simulink model "TestPath"  (R2022b)
settings: Solver=VariableStepAuto  StartTime=0.0  StopTime=1  RelTol=1e-3
settings Model: Creator=ADMIN  LastModifiedBy=ADMIN

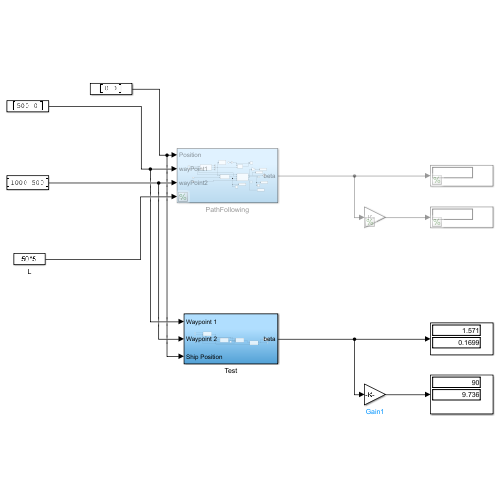
[thumbnail: Simulink's stored preview of the top-level diagram]
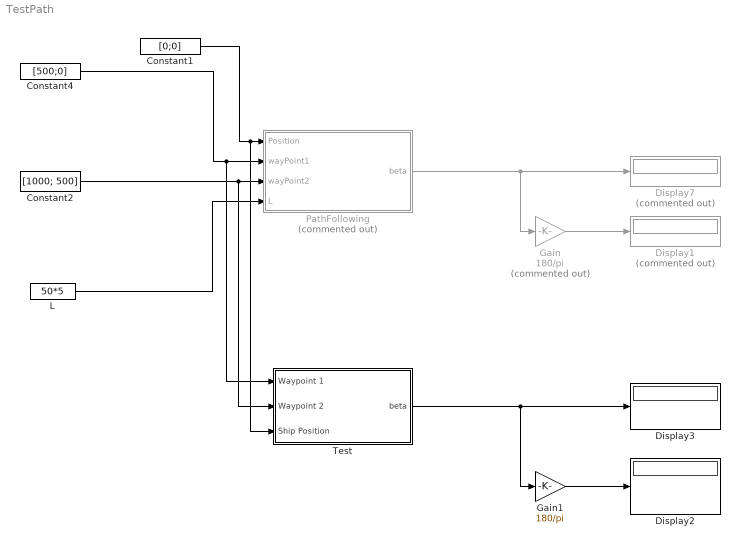
== system TestPath ==
  Constant1 : Constant  Value=[0;0]
  Constant2 : Constant  Value=[1000; 500]
  Constant4 : Constant  Value=[500;0]
  Display1 : Display  Commented=on
  Display2 : Display
  Display3 : Display
  Display7 : Display  Commented=on
  Gain : Gain  Commented=on  Gain=180/pi
  Gain1 : Gain  Gain=180/pi
  L : Constant  Value=50*5
  PathFollowing : Subsystem  Commented=on
  Test : Subsystem
  wires:
  PathFollowing/1(beta) -> Gain/1, Display7/1
  Constant2/1 -> PathFollowing/3(wayPoint2), Test/2(Waypoint 2)
  L/1 -> PathFollowing/4(L)
  Constant4/1 -> PathFollowing/2(wayPoint1), Test/1(Waypoint 1)
  Constant1/1 -> Test/3(Ship Position), PathFollowing/1(Position)
  Gain/1 -> Display1/1
  Gain1/1 -> Display2/1
  Test/1(beta) -> Display3/1, Gain1/1

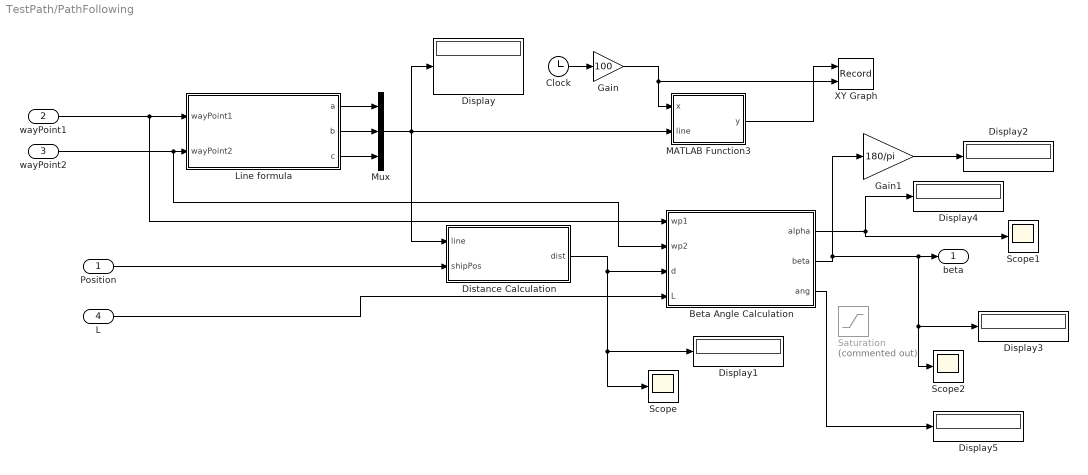
== system TestPath/PathFollowing ==
  Position : Inport
  wayPoint1 : Inport  Port=2
  wayPoint2 : Inport  Port=3
  L : Inport  Port=4
  Beta Angle Calculation : MATLAB Function  TreatAsAtomicUnit=on
  Clock : Clock
  Display{,1..5} (6 alike) : Display
  Distance Calculation : MATLAB Function  TreatAsAtomicUnit=on
  Gain : Gain  Gain=100
  Gain1 : Gain  Gain=180/pi
  Line formula : MATLAB Function  TreatAsAtomicUnit=on
  MATLAB Function3 : MATLAB Function  TreatAsAtomicUnit=on
  Mux : Mux  Inputs=3
  Saturation : Saturate  Commented=on
  Scope : Scope
  Scope1 : Scope
  Scope2 : Scope
  XY Graph : Record  FileSettingsInternal="{\"entries\":[{\"content\":{\"excelSettings\":{\"content\":{},\"type\":\"Streamout.ExcelSettings\"}},\"type\":\"Streamout.FileSettingStorage\",\"uuid\":\"7b3461a9-4dfd-4a0d-8e09-ea25a3eef10c\"}],\"packageUris\":[\"http://schema.mathworks.com/mf0/streamout_blocks/R2020a\"],\"version\":\"1.0\"}"  Layout=[1 1]  SignalsInternal="{\"entries\":[{\"content\":{\"signals\":[{\"content\":{\"blockPath\":[\"TestPath/PathFollowing/XY Graph\"],\"channel\":[],\"dimensions\":[1],\"domain\":\"TestPath/PathFollowing/XY Graph\",\"lineColor\":\"#64d413\",\"plots\":[1],\"port\":1,\"sid\":[],\"signalID\":197,\"signalName\":\"MATLAB Function3\"},\"type\":\"RecordBlkView.Signal\",\"uuid\":\"7b2fa58a-99ab-4b68-b3c2-9f07c173279a\"},{\"content\":{\"blockPath\":[\"TestPath/PathFollowing/XY Graph\"],\"channel\":[],\"dimensions\":[1],\"domain\":\"TestPath/PathFollowing/XY Graph\",\"lineColor\":\"#ff13a6\",\"plots\":[1],\"port\":2,\"sid\":[],\"signalID\":200,\"signalName\":\"Gain\"},\"type\":\"RecordBlkView.Signal\",\"uuid\":\"ec02b214-b15a-4d30-961c-c4cd029c4cfa\"}]},\"type\":\"RecordBlkView.InputSignals\",\"uuid\":\"04f76249-43da-41fc-9b1b-82b52f6b110f\"}],\"packageUris\":[\"http://schema.mathworks.com/mf0/streamout_blocks/R2020a\"],\"version\":\"1.0\"}"  VisualizationBindings="{\"xyplotplugin\":{\"info\":[{\"series\":[{\"bindingParametersList\":[{\"parameter\":\"X-Axis\",\"signalID\":197,\"signalName\":\"MATLAB Function3\"},{\"parameter\":\"Y-Axis\",\"signalID\":200,\"signalName\":\"Gain\"}],\"seriesID\":38097}],\"subplotID\":1}]}}"  CompatibilityTag=XY
  beta : Outport
  wires:
  Line formula/2(b) -> Mux/2
  Line formula/1(a) -> Mux/1
  Line formula/3(c) -> Mux/3
  wayPoint1/1 -> Line formula/1(wayPoint1), Beta Angle Calculation/1(wp1)
  wayPoint2/1 -> Beta Angle Calculation/2(wp2), Line formula/2(wayPoint2)
  Mux/1 -> Distance Calculation/1(line), MATLAB Function3/2(line), Display/1
  Position/1 -> Distance Calculation/2(shipPos)
  Distance Calculation/1(dist) -> Display1/1, Scope/1, Beta Angle Calculation/3(d)
  L/1 -> Beta Angle Calculation/4(L)
  Beta Angle Calculation/2(beta) -> Scope2/1, Display3/1, beta/1, Gain1/1
  Gain1/1 -> Display2/1
  Clock/1 -> Gain/1
  MATLAB Function3/1(y) -> XY Graph/1
  Gain/1 -> XY Graph/2, MATLAB Function3/1(x)
  Beta Angle Calculation/1(alpha) -> Display4/1, Scope1/1
  Beta Angle Calculation/3(ang) -> Display5/1

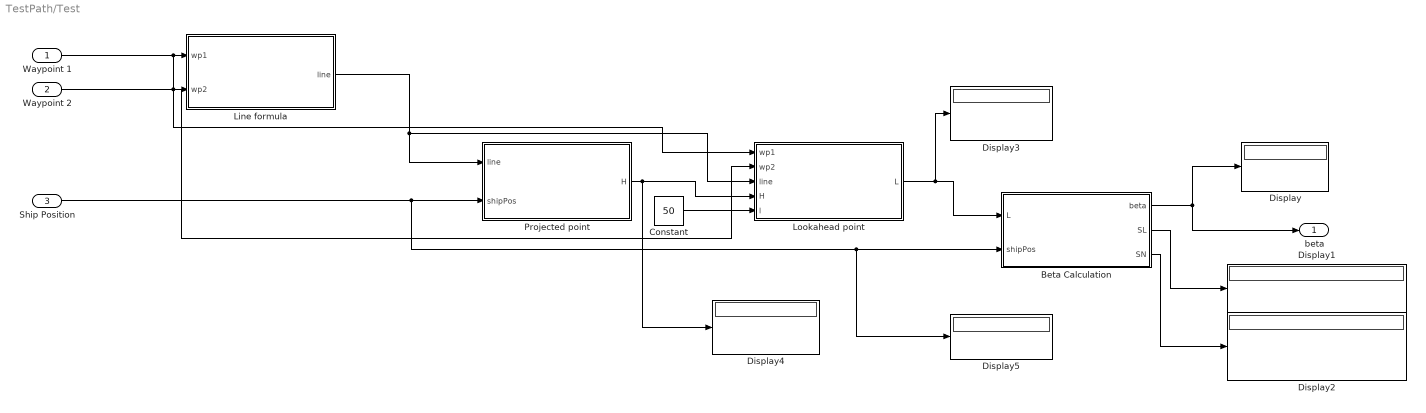
== system TestPath/Test ==
  Waypoint 1 : Inport
  Waypoint 2 : Inport  Port=2
  Ship Position : Inport  Port=3
  Beta Calculation : MATLAB Function  TreatAsAtomicUnit=on
  Constant : Constant  Value=50
  Display{,1..5} (6 alike) : Display
  Line formula : MATLAB Function  TreatAsAtomicUnit=on
  Lookahead point : MATLAB Function  TreatAsAtomicUnit=on
  Projected point : MATLAB Function  TreatAsAtomicUnit=on
  beta : Outport
  wires:
  Waypoint 1/1 -> Lookahead point/1(wp1), Line formula/1(wp1)
  Waypoint 2/1 -> Lookahead point/2(wp2), Line formula/2(wp2)
  Line formula/1(line) -> Lookahead point/3(line), Projected point/1(line)
  Ship Position/1 -> Projected point/2(shipPos), Display5/1, Beta Calculation/2(shipPos)
  Projected point/1(H) -> Display4/1, Lookahead point/4(H)
  Constant/1 -> Lookahead point/5(l)
  Lookahead point/1(L) -> Display3/1, Beta Calculation/1(L)
  Beta Calculation/1(beta) -> beta/1, Display/1
  Beta Calculation/2(SL) -> Display1/1
  Beta Calculation/3(SN) -> Display2/1

== matlab function TestPath/Test/Line formula ==
  data: wp1 input; line output; wp2 input
function line = fcn(wp1, wp2)

% Reverse coordinate of points
wayPoint1 = flip(wp1);
wayPoint2 = flip(wp2);

a = (wayPoint2(1) - wayPoint1(1)) / (wayPoint2(2) - wayPoint1(2));
b = -1;
c = wayPoint1(2) - a*wayPoint1(1);

line = [a, b, c];
% ax + by + c = 0

== matlab function TestPath/Test/Projected point ==
  data: line input; H output; shipPos input
function H = fcn(line, shipPos) 
coder.extrinsic('PointProjection');
H = [0, 0];
H = PointProjection(shipPos, line);

== matlab function TestPath/Test/Lookahead point ==
  data: wp1 input; wp2 input; line input; L output; H input; l input
function L = fcn(wp1, wp2, line, H, l)
lineFormula = line;
projectedPoint = H;
distance = l;
coder.extrinsic('LookAhead');
L = [0 0];
L = LookAhead(wp1, wp2, lineFormula, projectedPoint, distance);

== matlab function TestPath/Test/Beta Calculation ==
  data: L input; beta output; shipPos input; SL output; SN output
function [beta, SL, SN] = fcn(L, shipPos)

N = shipPos' + [0 500]; % arbitrary point on the North axis of the ship
SL = L - shipPos'; % lookahead vector
SN = N - shipPos'; % North vector
beta = acos(dot(SL, SN) / (norm(SL) * norm(SN))); % angle between 2 vectors

% Determine correct sign for beta
if L(1) < shipPos(1)
   beta = -beta;
end

== matlab function TestPath/PathFollowing/Line formula ==
  data: wayPoint1 input; a output; wayPoint2 input; b output; c output
function [a,b,c] = fcn(wayPoint1, wayPoint2)

a = (wayPoint2(1) - wayPoint1(1)) / (wayPoint2(2) - wayPoint1(2));
b = -1;
c = wayPoint1(2) - a*wayPoint1(1);

% ax + by + c = 0

== matlab function TestPath/PathFollowing/Distance Calculation ==
  data: line input; dist output; shipPos input
function dist = fcn(line,shipPos)

dist = abs(line(1)*shipPos(1) + line(2)*shipPos(2) + line(3)) / sqrt(line(1)^2 + line(2)^2);

% d = |ax+by+c|/sqrt(a^2 + b^2)

== matlab function TestPath/PathFollowing/Beta Angle Calculation ==
  data: alpha output; wp1 input; wp2 input; d input; beta output; L input; ang output
function [alpha, beta, ang] = BetaCal(wp1, wp2, d, L)

% line coefficient
alpha = atan2((wp2(1) - wp1(1)) , (wp2(2) - wp1(2)));
% ax+by+c=0

beta = atan2(L,d) - alpha;
ang = atan2(L,d);

== matlab function TestPath/PathFollowing/MATLAB Function3 ==
  data: x input; y output; line input
function y = fcn(x,line)

y = line(1)*x+line(3);
